simulink model "OVF2D"  (R2022b)
settings: Solver=FixedStepAuto  StartTime=0.0  StopTime=15  FixedStep=ts  MaxStep=0.6  RelTol=1e-3
values from neighbouring files (symbols this model uses):
  N = 4    [OVFMain.m]
  p_obstacle = [2,3;3,7;7.5,5.5]    [OVFMain.m]
  p_target = [9,10;3,10;6,10;0,10]    [OVFMain.m]
  ra = 0.6    [OVFMain.m]
  ro = [1.3;1.4;1.8]    [OVFMain.m]
  rs = 0.4    [OVFMain.m]
  v_max = 2    [OVFMain.m]
  v_max1 = 20    [OVFMain.m]
libraries: aerolibanimutils x1
settings Model: Creator=51078  LastModifiedBy=51078
settings SolverCC: AlgebraicLoopSolver=TrustRegion
settings DataIOCC: ReturnWorkspaceOutputs=off
settings DebuggingCC: UnconnectedInputMsg=warning  UnconnectedOutputMsg=warning  UnconnectedLineMsg=warning  SFMachineParentedDataDiag=warning  ArithmeticOperatorsInVariantConditions=warning
settings ModelReferenceCC: EnableRefExpFcnMdlSchedulingChecks=on
settings SFSimCC: SimUseLocalCustomCode=off  CustomCodeUndefinedFunction=UseInterfaceOnly
settings RTWCC: RTWUseLocalCustomCode=off  DLArmComputeVersion=19.05
settings CodeAppCC: StateflowObjectComments=on

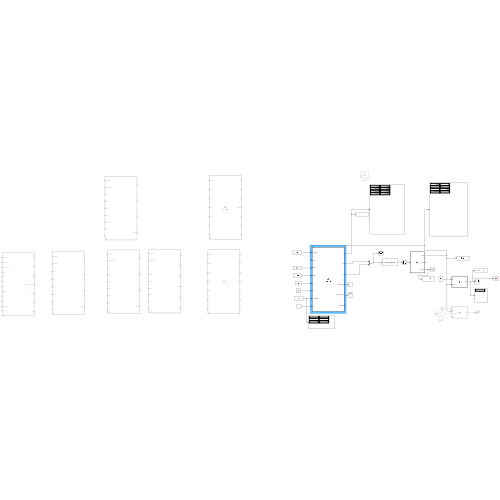
[thumbnail: Simulink's stored preview of the top-level diagram]
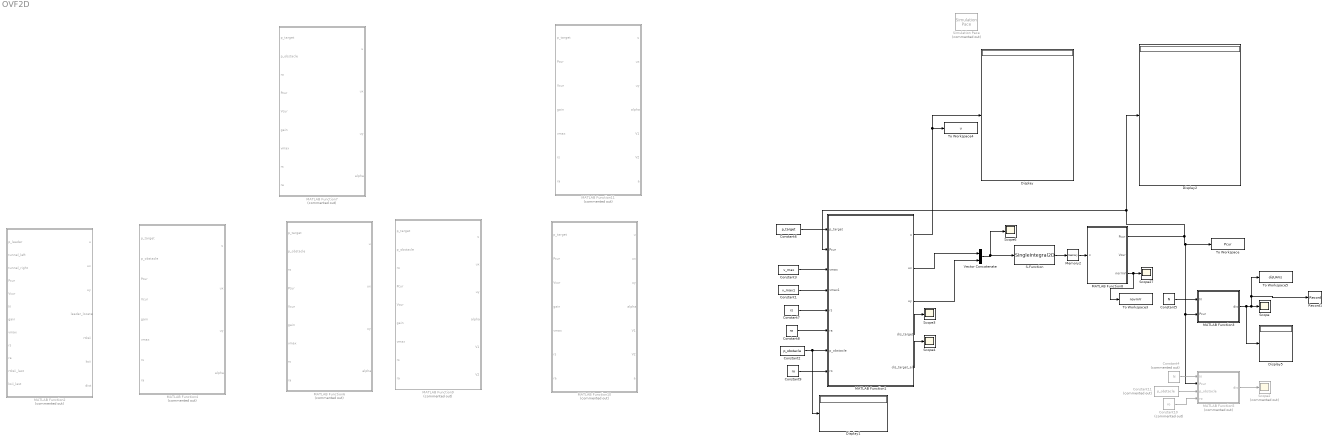
== system OVF2D ==
  Constant1 : Constant  Value=v_max1
  Constant10 : Constant  Commented=on  Value=ro
  Constant11 : Constant  Commented=on  Value=p_obstacle
  Constant2 : Constant  Value=p_obstacle
  Constant3 : Constant  Value=v_max
  Constant4 : Constant  Commented=on  Value=N
  Constant5 : Constant  Value=N
  Constant6 : Constant  Value=p_target
  Constant7 : Constant  Value=rs
  Constant8 : Constant  Value=ra
  Constant9 : Constant  Value=ro
  Display{,1..2,5} (4 alike) : Display
  MATLAB Function1 : MATLAB Function  TreatAsAtomicUnit=on
  MATLAB Function10 : MATLAB Function  Commented=on  TreatAsAtomicUnit=on
  MATLAB Function11 : MATLAB Function  Commented=on  TreatAsAtomicUnit=on
  MATLAB Function2 : MATLAB Function  Commented=on  TreatAsAtomicUnit=on
  MATLAB Function3 : MATLAB Function  TreatAsAtomicUnit=on
  MATLAB Function4 : MATLAB Function  Commented=on  TreatAsAtomicUnit=on
  MATLAB Function5 : MATLAB Function  Commented=on  TreatAsAtomicUnit=on
  MATLAB Function6 : MATLAB Function  Commented=on  TreatAsAtomicUnit=on
  MATLAB Function7 : MATLAB Function  Commented=on  TreatAsAtomicUnit=on
  MATLAB Function8 : MATLAB Function  TreatAsAtomicUnit=on
  MATLAB Function9 : MATLAB Function  Commented=on  TreatAsAtomicUnit=on
  Memory2 : Memory
  Record1 : Record  FileSettingsInternal="{\"entries\":[{\"content\":{\"excelSettings\":{\"content\":{},\"type\":\"Streamout.ExcelSettings\"}},\"type\":\"Streamout.FileSettingStorage\",\"uuid\":\"113e7f0b-c50f-4f8c-84db-ec7da5fa2ec4\"}],\"packageUris\":[\"http://schema.mathworks.com/mf0/streamout_blocks/R2020a\"],\"version\":\"1.0\"}"  Layout=[1 1]  SignalsInternal="{\"entries\":[{\"content\":{\"signals\":[{\"content\":{\"blockPath\":[\"OVF2D/Record1\"],\"channel\":[],\"dimensions\":[1],\"domain\":\"OVF2D/Record1\",\"lineColor\":\"#d95319\",\"plots\":[],\"port\":1,\"sid\":[\"\"],\"signalID\":16,\"signalName\":\"MATLAB Function3\"},\"type\":\"RecordBlkView.Signal\",\"uuid\":\"cb360406-dc3a-4a23-b0a4-c1b09b6a15ae\"}]},\"type\":\"RecordBlkView.InputSignals\",\"uuid\":\"8c052846-9eb7-4e55-9645-09fc1fafe585\"}],\"packageUris\":[\"http://schema.mathworks.com/mf0/streamout_blocks/R2020a\"],\"version\":\"1.0\"}"  VisualizationBindings="{\"sparklinesplugin\":{\"info\":[{\"bindingParametersList\":[],\"subplotID\":1}]}}"
  S-Function : S-Function  FunctionName=SingleIntegral2D  SFunctionDeploymentMode=off  EnableBusSupport=off
  Scope{,3..4,6,27} (5 alike) : Scope
  Scope2 : Scope  Commented=on
  Simulation Pace : aerolibanimutils/Simulation Pace  Commented=on  SimulationPace=1  SleepMode=MATLAB Thread  OutputPaceError=off  SampleTime=0.01
  To Workspace : ToWorkspace  VariableName=Pcur  SaveFormat=Timeseries  SampleTime=-1
  To Workspace3 : ToWorkspace  VariableName=novmV  SaveFormat=Timeseries  SampleTime=-1
  To Workspace4 : ToWorkspace  VariableName=u  SaveFormat=Timeseries  SampleTime=-1
  To Workspace5 : ToWorkspace  VariableName=disUAVs  SaveFormat=Timeseries  SampleTime=-1
  Vector Concatenate : Concatenate
  wires:
  Constant3/1 -> MATLAB Function1/3(vmax)
  Constant7/1 -> MATLAB Function1/5(rs)
  Constant8/1 -> MATLAB Function1/6(ra)
  MATLAB Function1/1(u) -> Display/1, To Workspace4/1
  Constant5/1 -> MATLAB Function3/1(N)
  MATLAB Function3/1(dis) -> Display5/1, Scope/1, Record1/1, To Workspace5/1
  Constant6/1 -> MATLAB Function1/1(p_target)
  MATLAB Function1/2(ux) -> Vector Concatenate/1
  MATLAB Function1/3(uy) -> Vector Concatenate/2
  MATLAB Function8/3(normV) -> To Workspace3/1, Scope27/1
  MATLAB Function8/1(Pcur) -> MATLAB Function5/2(Pcur), MATLAB Function3/2(Pcur), To Workspace/1, Display2/1, MATLAB Function1/2(Pcur)
  S-Function/1 -> Memory2/1
  Constant4/1 -> MATLAB Function5/1(N)
  MATLAB Function5/1(dis) -> Scope2/1
  Constant10/1 -> MATLAB Function5/4(ro)
  Constant11/1 -> MATLAB Function5/3(p_obstacle)
  MATLAB Function1/4(dis_target) -> Scope3/1
  Vector Concatenate/1 -> Scope6/1, S-Function/1
  Memory2/1 -> MATLAB Function8/1(x)
  Constant1/1 -> MATLAB Function1/4(vmax1)
  Constant2/1 -> Display1/1, MATLAB Function1/7(p_obstacle)
  Constant9/1 -> MATLAB Function1/8(ro)
  MATLAB Function1/5(dis_target_all) -> Scope4/1

== matlab function OVF2D/MATLAB Function6 ==
  data: p_target input; p_obstacle input; ro input; u output size=[N,2]; ux output size=[N,1]; uy output size=[N,1]; Pcur input; Vcur input; gain input; vmax input; rs input; ra input; alpha output
function [u,ux,uy,alpha]  = mytunnel(p_target,p_obstacle,ro,Pcur,Vcur,gain,vmax,rs,ra)
N=1;

e1=zeros(N,2);
V1=zeros(N,2);
V2=zeros(N,2);
V3=zeros(N,2);
V=zeros(N,2);

u=zeros(N,2);
ux=zeros(N,1);
uy=zeros(N,1);
OVF=2*ones(N,1);
alpha=zeros(N,1);

k1=1;
k2=40;
v2=zeros(N,2);
for i=1:N
    v_line=vmax;
    e1(i,:) = (p_target(i,:)-(Pcur(i,:)+1/gain*Vcur(i,1:2)))/norm(p_target(i,:)-(Pcur(i,:)+1/gain*Vcur(i,1:2)))*(v_line);
    V1(i,:) = mysat(k1*e1(i,:),vmax);
    
    for j=1:N
        if i~=j
            em = 0;
            ksimil = (Pcur(i,1:2) - Pcur(j,1:2)) + 1/gain*(Vcur(i,1:2) - Vcur(j,1:2));
            bil = k2*dmysigma2(norm(ksimil),2*rs,rs+ra,em);
            v2(i,:) = v2(i,:) + bil*(ksimil/norm(ksimil));
        end
    end
    
    for k=1:length(ro)
        em = 0;
        ksimik = (Pcur(i,1:2) - p_obstacle(k,1:2)) + 1/gain*(Vcur(i,1:2));
        bil = k2*dmysigma2(norm(ksimik),rs+ro(i),ro(i)+ra,em);
        v2(i,:) = v2(i,:) + bil*(ksimik/norm(ksimik));       
    end
    if isnan(v2(i,1)) || isnan(v2(i,2))
        v2(i,:)=[0,0];
    end
    
    
    
    ksiwp=(p_target(i,:)-(Pcur(i,:)+1/gain*Vcur(i,1:2)))/norm(p_target(i,:)-(Pcur(i,:)+1/gain*Vcur(i,1:2)));
    Ai = ksiwp'*ksiwp;    
    a=dot(v2(i,:),ksiwp)/(norm(v2(i,:))*norm(ksiwp));
    costheta1=-2/sqrt(5);
    costheta2=(norm(V1(i,:))-sqrt(5*norm(V1(i,:))^2+4*norm(v2(i,:))^2))/(2*norm(v2(i,:)));
    alpha(i)=mysigma3(a,costheta2,costheta1);
%     if a>0
%         alpha(i)=0;
%     end
     V2(i,:) = ((eye(2)-alpha(i)*Ai)*v2(i,:)')';

    % V2(i,:)=v2(i,:);
     
    if isnan(V2(i,1)) || isnan(V2(i,2))
        V2(i,:)=[0,0];
    end
    
    V(i,:)=mysat(V1(i,:)+V2(i,:),vmax);
end


u=V;
ux = u(:,1);
uy = u(:,2);

== matlab function OVF2D/MATLAB Function7 ==
  data: p_target input; p_obstacle input; ro input; u output size=[N,2]; ux output size=[N,1]; uy output size=[N,1]; Pcur input; Vcur input; gain input; vmax input; rs input; ra input; alpha output
function [u,ux,uy,alpha]  = mytunnel(p_target,p_obstacle,ro,Pcur,Vcur,gain,vmax,rs,ra)
N=1;

e1=zeros(N,2);
V1=zeros(N,2);
V2=zeros(N,2);
V3=zeros(N,2);
V=zeros(N,2);

u=zeros(N,2);
ux=zeros(N,1);
uy=zeros(N,1);
OVF=2*ones(N,1);
alpha=zeros(N,1);

k1=1;
k2=4;
v2=zeros(N,2);
for i=1:N
    v_line=vmax;
    e1(i,:) = (p_target(i,:)-(Pcur(i,:)+1/gain*Vcur(i,1:2)))/norm(p_target(i,:)-(Pcur(i,:)+1/gain*Vcur(i,1:2)))*(v_line);
    V1(i,:) = mysat(k1*e1(i,:),vmax);
    
    for j=1:N
        if i~=j
            em = 0;
            ksimil = (Pcur(i,1:2) - Pcur(j,1:2)) + 1/gain*(Vcur(i,1:2) - Vcur(j,1:2));
            bil = k2*dmysigma2(norm(ksimil),2*rs,rs+ra,em);
            v2(i,:) = v2(i,:) + bil*(ksimil/norm(ksimil));
        end
    end
    
    for k=1:length(ro)
        em = 0;
        ksimik = (Pcur(i,1:2) - p_obstacle(k,1:2)) + 1/gain*(Vcur(i,1:2));
        
%         bil = k2*dmysigma2(norm(ksimik),rs+ro(i),ro(i)+ra,em);
%         v2(i,:) = bil*(ksimik/norm(ksimik));     

        v2(i,:) = k2*norm((Pcur(i,:)+1/gain*Vcur(i,1:2))-p_target(i,:))^2*dmysigma2(norm(ksimik),rs+ro(i),ro(i)+ra,em)*(ksimik/norm(ksimik))...
            +mysigma2(norm(ksimik),rs+ro(i),ro(i)+ra,em)*2*(p_target(i,:)-(Pcur(i,:)+1/gain*Vcur(i,1:2)));     
        
        ksiwp=(p_target(i,:)-(Pcur(i,:)+1/gain*Vcur(i,1:2)))/norm(p_target(i,:)-(Pcur(i,:)+1/gain*Vcur(i,1:2)));
        Ai = ksiwp'*ksiwp;
        a=dot(v2(i,:),ksiwp)/(norm(v2(i,:))*norm(ksiwp));
        costheta1=-2/sqrt(5);
        costheta2=(norm(V1(i,:))-sqrt(5*norm(V1(i,:))^2+4*norm(v2(i,:))^2))/(2*norm(v2(i,:)));
        alpha(i)=mysigma3(a,costheta2,costheta1);
        %     if a>0
        %         alpha(i)=0;
        %     end
%         V2(i,:) = V2(i,:)+((eye(2)-alpha(i)*Ai)*v2(i,:)')';
         V2(i,:) = V2(i,:)+v2(i,:);

    end
    if isnan(V2(i,1)) || isnan(V2(i,2))
        V2(i,:)=[0,0];
    end
    
    V(i,:)=mysat(V1(i,:)+V2(i,:),vmax);
end


u=V;
ux = u(:,1);
uy = u(:,2);

== matlab function OVF2D/MATLAB Function2 ==
  data: p_leader input; tunnel_left input; u output size=[20,2]; ux output size=[20,1]; uy output size=[20,1]; tunnel_right input; Pcur input; Vcur input; N input; gain input; vmax input; leader_locate output; rs input; ra input; rtksii_last input; ksii_last input; rtksii output size=[20,1]; ksii output size=[20,2]; dist output
function [u,ux,uy,leader_locate,rtksii,ksii,dist]  = mytunnel(p_leader,tunnel_left,tunnel_right,Pcur,Vcur,N,gain,vmax,rs,ra,rtksii_last,ksii_last)

leader_locate=zeros(20,1);
for i=1:N
    dis_leader_min=10^8;
    for j=1:length(p_leader(:,1))
        dis_leader=norm(Pcur(i,:)-p_leader(j,:));
        if dis_leader < dis_leader_min
            leader_locate(i)=j;
            dis_leader_min=dis_leader;
        end
    end
end

nc=zeros(length(tunnel_left(:,1)),2);
for i=1:length(tunnel_left(:,1))
    rot=[0 -1;1 0]; %逆时针90度
    C=rot*(tunnel_right(i,:)-tunnel_left(i,:))';
    nc(i,:)=-(C/norm(C))';
end

e1=zeros(N,2);
V1=zeros(N,2);
V2=zeros(N,2);
V3=zeros(N,2);
V=zeros(N,2);

u=zeros(20,2);
ux=zeros(20,1);
uy=zeros(20,1);

rtksii=zeros(20,1);
ksiti=zeros(20,2);
ksii=zeros(20,2);
pti=zeros(20,2);

dis=10^5;
dist=10^5;


rs1=rs;
v_line=0;
for i=1:N
    if leader_locate(i)~=0
%         if i>=1 && i<=5
%             v_line=vmax;
%         elseif i>=6 && i<=10
%             v_line=vmax-0.7;
%         elseif i>=11 && i<=15
%             v_line=vmax-1.4;
%         elseif i>=16 && i<=20
%             v_line=vmax-2.1;
%         end
        v_line=vmax;
        
        %v_line=0.5*vmax;
        k1=1;
        e1(i,:) = nc(leader_locate(i),:)*(v_line);
        V1(i,:) = -mysat(k1*e1(i,:),vmax);
        
        et=10^(-1);e = 0.000001;
        k3=1;
        mksii=0.5*(tunnel_left(leader_locate(i),:)+tunnel_right(leader_locate(i),:));
        ksii(i,:) = Pcur(i,1:2) + 1/gain*Vcur(i,1:2);
        ksiti(i,:) = Pcur(i,1:2) + 1/gain*Vcur(i,1:2) - mksii;
        rtksii(i)=0.5*norm(tunnel_left(leader_locate(i),:)-tunnel_right(leader_locate(i),:));
        
        pti(i,:)= Pcur(i,1:2) - mksii;
        disti =  rtksii(i) - norm(pti(i,:));
        if disti<dist
            dist=disti;
        end
        
        temp_t=(rtksii(i)-rs1)-norm(ksiti(i,:))*mys((rtksii(i)-rs1)/(norm(ksiti(i,:))+et),e);
        dVtidksiti=(-k3*dmysigma(rtksii(i)-norm(ksiti(i,:)),rs1,ra)*temp_t+k3*mysigma(rtksii(i)-norm(ksiti(i,:)),rs1,ra)*(mys((rtksii(i)-rs1)/(norm(ksiti(i,:))+et),e)-norm(ksiti(i,:))*(rtksii(i)-rs1)/((norm(ksiti(i,:))+et)^2)*dmys((rtksii(i)-rs1)/(norm(ksiti(i,:))+et),e)))/(temp_t^2);
        dVtidrtksii=(k3*dmysigma(rtksii(i)-norm(ksiti(i,:)),rs1,ra)*temp_t-k3*mysigma(rtksii(i)-norm(ksiti(i,:)),rs1,ra)*(1-(norm(ksiti(i,:))/(norm(ksiti(i,:))+et))*dmys((rtksii(i)-rs1)/(norm(ksiti(i,:))+et),e)))/(temp_t^2);
        if ksii(i,1)-ksii_last(i,1)==0 || ksii(i,2)-ksii_last(i,2)==0
            drtpdksii=[0,0];
        else
            drtpdksii=[(rtksii(i)-rtksii_last(i))/(ksii(i,1)-ksii_last(i,1)),(rtksii(i)-rtksii_last(i))/(ksii(i,2)-ksii_last(i,2))];
        end
        ci=dVtidksiti*ksiti(i,:)/norm(ksiti(i,:))+dVtidrtksii*drtpdksii;
        
        un=ksiti(i,:)-(dot(ksiti(i,:),nc(leader_locate(i),:))*nc(leader_locate(i),:));
        V3(i,:)=-(un/norm(un))*dot(un/norm(un),ci);
        if isnan(V3(i,1)) || isnan(V3(i,2))
            V3(i,:)=[0,0];
        end
    end
    
    for j=1:N
        if i~=j
            k2 = 1; e = 0.000001;
            ksimil = (Pcur(i,1:2) - Pcur(j,1:2)) + 1/gain*(Vcur(i,1:2) - Vcur(j,1:2));
            temp = (1+e)*norm(ksimil) - (2*rs)*mys(norm(ksimil)/(2*rs),e);
            bil = k2*dmysigma(norm(ksimil),2*rs,rs+ra)/temp ...
                - k2*mysigma(norm(ksimil),2*rs,rs+ra)*((1+e)-dmys(norm(ksimil)/(2*rs),e))/(temp^2);
            V2(i,:) = V2(i,:)- bil*(ksimil/norm(ksimil));
            if isnan(V2(i,1)) || isnan(V2(i,2))
                V2(i,:)=[0,0];
            end
            disij=norm(Pcur(i,1:2) - Pcur(j,1:2));
            if disij<dis
                dis=disij;
            end
        end
    end
    V(i,:)=mysat(V1(i,:)+V2(i,:)+V3(i,:),vmax);
end
% V11=[V1(1,1:2);V1(2,1:2);V1(3,1:2);V1(4,1:2)];
% V21=[V2(1,1:2);V2(2,1:2);V2(3,1:2);V2(4,1:2)];
% V31=[V3(1,1:2);V3(2,1:2);V3(3,1:2);V3(4,1:2)];



u = [V(1,1:2);V(2,1:2);V(3,1:2);V(4,1:2);V(5,1:2);V(6,1:2);V(7,1:2);V(8,1:2);V(9,1:2);V(10,1:2);V(11,1:2);V(12,1:2);V(13,1:2);V(14,1:2);V(15,1:2);V(16,1:2);V(17,1:2);V(18,1:2);V(19,1:2);V(20,1:2)];
ux = u(:,1);
uy = u(:,2);

== matlab function OVF2D/MATLAB Function9 ==
  data: p_target input; p_obstacle input; ro input; u output size=[N,2]; ux output size=[N,1]; uy output size=[N,1]; Pcur input; Vcur input; gain input; vmax input; rs input; ra input; alpha output; V1 output; V2 output
function [u,ux,uy,alpha,V1,V2]  = mytunnel(p_target,p_obstacle,ro,Pcur,Vcur,gain,vmax,rs,ra)
tic
N=1;

e1=zeros(N,2);
V1=zeros(N,2);
V2=zeros(N,2);
V3=zeros(N,2);
V=zeros(N,2);

u=zeros(N,2);
ux=zeros(N,1);
uy=zeros(N,1);
OVF=2*ones(N,1);
alpha=zeros(N,1);

k1=1;
k2=4;
v2=zeros(N,2);
for i=1:N
    v_line=vmax;
    e1(i,:) = (p_target(i,:)-(Pcur(i,:)+1/gain*Vcur(i,1:2)))/norm(p_target(i,:)-(Pcur(i,:)+1/gain*Vcur(i,1:2)))*(v_line);
    V1(i,:) = mysat(k1*e1(i,:),vmax);
    
    for j=1:N
        if i~=j
            em = 0;
            ksimil = (Pcur(i,1:2) - Pcur(j,1:2)) + 1/gain*(Vcur(i,1:2) - Vcur(j,1:2));
            bil = k2*dmysigma2(norm(ksimil),2*rs,rs+ra,em);
            v2(i,:) = v2(i,:) + bil*(ksimil/norm(ksimil));
        end
    end
    
    for k=1:length(ro)
        em = 0;
        ksimik = (Pcur(i,1:2) - p_obstacle(k,1:2)) + 1/gain*(Vcur(i,1:2));
        
        bil = k2*dmysigma2(norm(ksimik),rs+ro(i),ro(i)+ra,em);
        v2(i,:) = bil*(ksimik/norm(ksimik));     
       
        ksiwp=(p_target(i,:)-(Pcur(i,:)+1/gain*Vcur(i,1:2)))/norm(p_target(i,:)-(Pcur(i,:)+1/gain*Vcur(i,1:2)));
        Ai = ksiwp'*ksiwp;
        a=dot(v2(i,:),ksiwp)/(norm(v2(i,:))*norm(ksiwp));
        costheta1=-2/sqrt(5);
        costheta2=(norm(V1(i,:))-sqrt(5*norm(V1(i,:))^2+4*norm(v2(i,:))^2))/(2*norm(v2(i,:)));
        alpha(i)=mysigma3(a,costheta2,costheta1);
        %     if a>0
        %         alpha(i)=0;
        %     end
        
        V2(i,:) = V2(i,:)+((eye(2)-alpha(i)*Ai)*v2(i,:)')';
         %V2(i,:) = V2(i,:)+((eye(2)-Ai)*v2(i,:)')';

        %V2(i,:) = V2(i,:)+v2(i,:);

    end
    if isnan(V2(i,1)) || isnan(V2(i,2))
        V2(i,:)=[0,0];
    end
    
    V(i,:)=mysat(V1(i,:)+V2(i,:),vmax);
end


u=V;
ux = u(:,1);
uy = u(:,2);
toc

== matlab function OVF2D/MATLAB Function10 ==
  data: p_target input; u output size=[N,2]; ux output size=[N,1]; uy output size=[N,1]; Pcur input; Vcur input; gain input; vmax input; rs input; ra input; alpha output; V1 output; V2 output; a output
function [u,ux,uy,alpha,V1,V2,a]  = mytunnel(p_target,Pcur,Vcur,gain,vmax,rs,ra)
% p_obstacle=p_obstacle';
% p_target=p_target';

N=4;
a=zeros(N,1);

e1=zeros(N,2);
V1=zeros(N,2);
V2=zeros(N,2);
V3=zeros(N,2);
V=zeros(N,2);

u=zeros(N,2);
ux=zeros(N,1);
uy=zeros(N,1);
OVF=2*ones(N,1);
alpha=zeros(N,1);

k1=1;
k2=100;
k3=3;
v2=zeros(N,2);
Ai=zeros(2,2);

for i=1:N
    v_line=vmax;
    e1(i,:) = (p_target(i,:)-Pcur(i,:))/norm(p_target(i,:)-Pcur(i,:))*(v_line);
%     e1(i,:) = (p_target(i,:)-Pcur(i,:));
    V1(i,:) = mysat(k1*e1(i,:),vmax);
    
    for j=1:N
        if i~=j
%             em = 0;
%             ksimil = (Pcur(i,1:2) - Pcur(j,1:2));
%             bil = k2*dmysigma2(norm(ksimil),2*rs,rs+ra,em);
%             v2(i,:) = v2(i,:) + bil*(ksimil/norm(ksimil));
            e = 0.000001;
            ksimil =  Pcur(i,1:2) - Pcur(j,1:2);
            temp = (1+e)*norm(ksimil) - (2*rs)*mys(norm(ksimil)/(2*rs),e);
            bil = k2*dmysigma(norm(ksimil),2*rs,rs+ra)/temp ...
                - k2*mysigma(norm(ksimil),2*rs,rs+ra)*((1+e)-dmys(norm(ksimil)/(2*rs),e))/(temp^2);
            v2(i,:)  = v2(i,:)  -  bil*(ksimil/norm(ksimil));
        end
    end
    
    
%     ksiwp=(p_target(i,:)-(Pcur(i,:)+1/gain*Vcur(i,1:2)))/norm(p_target(i,:)-(Pcur(i,:)+1/gain*Vcur(i,1:2)));
%     Ai = ksiwp'*ksiwp;
%     a=dot(v2(i,:),ksiwp)/(norm(v2(i,:))*norm(ksiwp));
%     costheta1=-2/sqrt(5);
%     costheta2=(norm(V1(i,:))-sqrt(5*norm(V1(i,:))^2+4*norm(v2(i,:))^2))/(2*norm(v2(i,:)));
%     alpha(i)=mysigma3(a,costheta2,costheta1);
%     if a>0
%         alpha(i)=0;
%     end
%     V2(i,:) = V2(i,:)+((eye(2)-alpha(i)*Ai)*v2(i,:)')';

    
     costheta=dot(V1(i,:) ,v2(i,:) )/(norm(V1(i,:) )*norm(v2(i,:) ));     
    if V1(i,1)*v2(i,2)-V1(i,2)*v2(i,1)>0 && costheta<0
        V2(i,:)= v2(i,:) + (norm(v2(i,:))/(sqrt(1-costheta^2)/-costheta))*(Rotation(-pi/2)*v2(i,:)'/norm(v2(i,:)))';
    elseif V1(i,1)*v2(i,2)-V1(i,2)*v2(i,1)<0 && costheta<0
        V2(i,:)= v2(i,:) + (norm(v2(i,:))/(sqrt(1-costheta^2)/-costheta))*(Rotation(pi/2)*v2(i,:)'/norm(v2(i,:)))';
    elseif costheta>=0
        V2(i,:)= v2(i,:) ;
    elseif V1(i,1)*v2(i,2)-V1(i,2)*v2(i,1)==0 && costheta<0
        V2(i,:)= v2(i,:)+ (Rotation(pi/2)*v2(i,:)')';
    else
        V2(i,:)=zeros(1,2);
    end
    


    Ai = V1(i,:)'*V1(i,:)/(norm(V1(i,:))^2);
    costheta1=cos(deg2rad(125));
    costheta2=-sqrt(2)/2;
    alpha(i)=mysigma3(costheta,costheta2,costheta1);
    if costheta>0
        alpha(i)=0;
    end

    a(i)=V1(i,1)*v2(i,2)-V1(i,2)*v2(i,1);
    if V1(i,1)*v2(i,2)-V1(i,2)*v2(i,1)>0
        V3(i,:)= ((eye(2)-alpha(i)*Ai)*v2(i,:)')' + dmysigma2(costheta,-1,costheta2,0)*(Rotation(-pi/2)*v2(i,:)')';
    elseif V1(i,1)*v2(i,2)-V1(i,2)*v2(i,1)<0
        V3(i,:)= ((eye(2)-alpha(i)*Ai)*v2(i,:)')' + dmysigma2(costheta,-1,costheta2,0)*(Rotation(pi/2)*v2(i,:)')';
    elseif V1(i,1)*v2(i,2)-V1(i,2)*v2(i,1)==0 && costheta>0
        V3(i,:)= ((eye(2)-alpha(i)*Ai)*v2(i,:)')';
    elseif V1(i,1)*v2(i,2)-V1(i,2)*v2(i,1)==0 && costheta<0
        V3(i,:)= ((eye(2)-alpha(i)*Ai)*v2(i,:)')'+ dmysigma2(costheta,-1,costheta2,0)*(Rotation(pi/2)*v2(i,:)')';
    else
        V3(i,:)=zeros(1,2);
    end

%     V(i,:)=mysat(V1(i,:)+V3(i,:),vmax);
    V(i,:)=vmax*(V1(i,:)+V3(i,:))/norm(V1(i,:)+V3(i,:));

    if isnan(V(i,1)) || isnan(V(i,2))
        V(i,:)=[0,0];
    end
end


u=V;
ux = u(:,1);
uy = u(:,2);

== matlab function OVF2D/MATLAB Function11 ==
  data: p_target input; u output size=[N,2]; ux output size=[N,1]; uy output size=[N,1]; Pcur input; Vcur input; gain input; vmax input; rs input; ra input; alpha output; V1 output; V2 output; a output
function [u,ux,uy,alpha,V1,V2,a]  = mytunnel(p_target,Pcur,Vcur,gain,vmax,rs,ra)
% p_obstacle=p_obstacle';
% p_target=p_target';

N=4;
a=zeros(N,1);

e1=zeros(N,2);
V1=zeros(N,2);
V2=zeros(N,2);
V3=zeros(N,2);
V=zeros(N,2);

u=zeros(N,2);
ux=zeros(N,1);
uy=zeros(N,1);
OVF=2*ones(N,1);
alpha=zeros(N,1);

k1=1;
k2=100;
k3=3;
v2=zeros(N,2);
Ai=zeros(2,2);

for i=1:N
    v_line=vmax;
    e1(i,:) = (p_target(i,:)-Pcur(i,:))/norm(p_target(i,:)-Pcur(i,:))*(v_line);
%     e1(i,:) = log(p_target(i,:)-Pcur(i,:));
    V1(i,:) = k1*e1(i,:);
    
    for j=1:N
        if i~=j
%             em = 0;
%             ksimil = (Pcur(i,1:2) - Pcur(j,1:2));
%             bil = k2*dmysigma2(norm(ksimil),2*rs,rs+ra,em);
%             v2(i,:) = v2(i,:) + bil*(ksimil/norm(ksimil));
%             e = 0.000001;
%             ksimil =  Pcur(i,1:2) - Pcur(j,1:2);
%             temp = (1+e)*norm(ksimil) - (2*rs)*mys(norm(ksimil)/(2*rs),e);
%             bil = k2*dmysigma(norm(ksimil),2*rs,rs+ra)/temp ...
%                 - k2*mysigma(norm(ksimil),2*rs,rs+ra)*((1+e)-dmys(norm(ksimil)/(2*rs),e))/(temp^2);
%             v2(i,:)  = v2(i,:)  -  bil*(ksimil/norm(ksimil));
                ksimil =  Pcur(i,1:2) - Pcur(j,1:2);
                bil=1/(norm(ksimil)-2*rs);
                v2(i,:)  = v2(i,:)  +  bil*(ksimil/norm(ksimil));
        end
    end
    V2(i,:)=v2(i,:);
    
%     ksiwp=(p_target(i,:)-(Pcur(i,:)+1/gain*Vcur(i,1:2)))/norm(p_target(i,:)-(Pcur(i,:)+1/gain*Vcur(i,1:2)));
%     Ai = ksiwp'*ksiwp;
%     a=dot(v2(i,:),ksiwp)/(norm(v2(i,:))*norm(ksiwp));
%     costheta1=-2/sqrt(5);
%     costheta2=(norm(V1(i,:))-sqrt(5*norm(V1(i,:))^2+4*norm(v2(i,:))^2))/(2*norm(v2(i,:)));
%     alpha(i)=mysigma3(a,costheta2,costheta1);
%     if a>0
%         alpha(i)=0;
%     end
%     V2(i,:) = V2(i,:)+((eye(2)-alpha(i)*Ai)*v2(i,:)')';

    
%      costheta=dot(V1(i,:) ,v2(i,:) )/(norm(V1(i,:) )*norm(v2(i,:) ));     
%     if V1(i,1)*v2(i,2)-V1(i,2)*v2(i,1)>0 && costheta<0
%         V2(i,:)= v2(i,:) + (norm(v2(i,:))/(sqrt(1-costheta^2)/-costheta))*(Rotation(-pi/2)*v2(i,:)'/norm(v2(i,:)))';
%     elseif V1(i,1)*v2(i,2)-V1(i,2)*v2(i,1)<0 && costheta<0
%         V2(i,:)= v2(i,:) + (norm(v2(i,:))/(sqrt(1-costheta^2)/-costheta))*(Rotation(pi/2)*v2(i,:)'/norm(v2(i,:)))';
%     elseif costheta>=0
%         V2(i,:)= v2(i,:) ;
%     elseif V1(i,1)*v2(i,2)-V1(i,2)*v2(i,1)==0 && costheta<0
%         V2(i,:)= v2(i,:)+ (Rotation(pi/2)*v2(i,:)')';
%     else
%         V2(i,:)=zeros(1,2);
%     end
%     
% 
% 
%     Ai = V1(i,:)'*V1(i,:)/(norm(V1(i,:))^2);
%     costheta1=cos(deg2rad(125));
%     costheta2=-sqrt(2)/2;
%     alpha(i)=mysigma3(costheta,costheta2,costheta1);
%     if costheta>0
%         alpha(i)=0;
%     end
% 
%     a(i)=V1(i,1)*v2(i,2)-V1(i,2)*v2(i,1);
%     if V1(i,1)*v2(i,2)-V1(i,2)*v2(i,1)>0
%         V3(i,:)= ((eye(2)-alpha(i)*Ai)*v2(i,:)')' + dmysigma2(costheta,-1,costheta2,0)*(Rotation(-pi/2)*v2(i,:)')';
%     elseif V1(i,1)*v2(i,2)-V1(i,2)*v2(i,1)<0
%         V3(i,:)= ((eye(2)-alpha(i)*Ai)*v2(i,:)')' + dmysigma2(costheta,-1,costheta2,0)*(Rotation(pi/2)*v2(i,:)')';
%     elseif V1(i,1)*v2(i,2)-V1(i,2)*v2(i,1)==0 && costheta>0
%         V3(i,:)= ((eye(2)-alpha(i)*Ai)*v2(i,:)')';
%     elseif V1(i,1)*v2(i,2)-V1(i,2)*v2(i,1)==0 && costheta<0
%         V3(i,:)= ((eye(2)-alpha(i)*Ai)*v2(i,:)')'+ dmysigma2(costheta,-1,costheta2,0)*(Rotation(pi/2)*v2(i,:)')';
%     else
%         V3(i,:)=zeros(1,2);
%     end

    V(i,:)=mysat(V1(i,:)+V2(i,:),vmax);
%     V(i,:)=vmax*(V1(i,:)+V2(i,:))/norm(V1(i,:)+V2(i,:));
%     V(i,:)=V1(i,:)+V2(i,:);

    if isnan(V(i,1)) || isnan(V(i,2))
        V(i,:)=[0,0];
    end
end


u=V;
ux = u(:,1);
uy = u(:,2);

== matlab function OVF2D/MATLAB Function3 ==
  data: dis output; N input; Pcur input
function dis = fcn(N, Pcur)
dis=10^5;
for i=1:N
    for j=1:N
        if i~=j
            disij=norm(Pcur(i,1:2) - Pcur(j,1:2));
            if disij<dis
                dis=disij;
            end
        end
    end
end

== matlab function OVF2D/MATLAB Function8 ==
  data: x input; Pcur output size=[N,2]; Vcur output size=[N,2]; normV output
function [Pcur,Vcur,normV] = fcn(x)
N=4;
Pcur=zeros(N,2);
Vcur=zeros(N,2);
normV=zeros(N,1);
for i=1:N
    Pcur(i,1)=x(i);
    Pcur(i,2)=x(i+N);
    Vcur(i,1)=x(i+2*N);
    Vcur(i,2)=x(i+3*N);
    normV(i)=norm(Vcur(i,:));
end
end

== matlab function OVF2D/MATLAB Function1 ==
  data: p_target input; u output size=[N,2]; ux output size=[N,1]; uy output size=[N,1]; Pcur input; vmax input; vmax1 input; rs input; ra input; dis_target output; dis_target_all output; p_obstacle input; ro input
function [u,ux,uy,dis_target,dis_target_all]  = OVF(p_target,Pcur,vmax,vmax1,rs,ra,p_obstacle,ro)
% p_obstacle=p_obstacle';
% p_target=p_target';

N=4;
item=3;

e1=zeros(N,2);
V1=zeros(N,2);
V2=zeros(N,2);
V=zeros(N,2);

u=zeros(N,2);
ux=zeros(N,1);
uy=zeros(N,1);
gamma=zeros(N,1);

k1=1;
k2=10;
v2=zeros(N,2);
v3=zeros(N,2);
v4=zeros(N,2);

Ai=zeros(2,2);

dis_target_all=zeros(N,1);
dis_target=10^5;

for i=1:N
    dis_target_all(i)=norm(Pcur(i,1:2)-p_target(i,:));
end
dis_target=max(dis_target_all);

for i=1:N
    v_line=vmax;
    e1(i,:) = (p_target(i,:)-Pcur(i,:))/norm(p_target(i,:)-Pcur(i,:))*(v_line);
    V1(i,:) = mysat(k1*e1(i,:),vmax);
    
    for j=1:N
        if i~=j
            e = 0.000001;
            ksimil =  Pcur(i,1:2) - Pcur(j,1:2);
            temp = (1+e)*norm(ksimil) - (2*rs)*mys(norm(ksimil)/(2*rs),e);
            bil = k2*dmysigma(norm(ksimil),2*rs,rs+ra)/temp ...
                - k2*mysigma(norm(ksimil),2*rs,rs+ra)*((1+e)-dmys(norm(ksimil)/(2*rs),e))/(temp^2);
            v3(i,:)  = v3(i,:)  -  bil*(ksimil/norm(ksimil));
        end
    end
    
    for j=1:length(p_obstacle(:,1))
        e = 0.000001;
        ksimil =  Pcur(i,1:2) - p_obstacle(j,1:2);
        temp = (1+e)*norm(ksimil) - (rs+ro(j))*mys(norm(ksimil)/(rs+ro(j)),e);
        bil = k2*dmysigma(norm(ksimil),rs+ro(j),ra+ro(j))/temp ...
            - k2*mysigma(norm(ksimil),rs+ro(j),ra+ro(j))*((1+e)-dmys(norm(ksimil)/(rs+ro(j)),e))/(temp^2);
        v4(i,:)  = v4(i,:)  -  bil*(ksimil/norm(ksimil));
    end
    
    v2(i,:)=v3(i,:)+ v4(i,:);
    alpha=(norm(V1(i,:))-sqrt(5*norm(V1(i,:))^2+4*norm(v2(i,:))^2))/(2*norm(v2(i,:)));
    beta=norm(V1(i,:))/vmax1-sqrt(norm(V1(i,:))^2*norm(v2(i,:))^2+4*vmax1*norm(V1(i,:))^2*norm(v2(i,:))+4*vmax1^2*norm(v2(i,:))^2)/(2*vmax1*norm(v2(i,:)));
    mu=0;
    if norm(v2(i,:))<vmax1
        mu=alpha;
    elseif norm(v2(i,:))>=vmax1
        mu=beta;
    end
    
    Ai = (V1(i,:)/norm(V1(i,:)))'*(V1(i,:)/norm(V1(i,:)));
    chi=dot(v2(i,:),V1(i,:))/(norm(v2(i,:))*norm(V1(i,:)));
    gamma(i)=mysigma3(chi,mu,-2/sqrt(5)*mu/alpha);
    
    if item==1
        V2(i,:)=v2(i,:);
    elseif item==2
        V2(i,:)=mysat(v2(i,:),vmax1);
    elseif item==3
        if chi>0
            gamma(i)=0;
        end
        V2(i,:)=((eye(2)-gamma(i)*Ai)*mysat(v2(i,:),vmax1)')';
    end
    
    if isnan(V1(i,1))
        V1(i,:)=[0,0];
    end
    if isnan(V2(i,2))
        V2(i,:)=[0,0];
    end
    V(i,:)=mysat(V1(i,:)+V2(i,:),vmax);
end


u=V;
ux = u(:,1);
uy = u(:,2);

== matlab function OVF2D/MATLAB Function4 ==
  data: p_target input; p_obstacle input; u output size=[N,2]; ux output size=[N,1]; uy output size=[N,1]; Pcur input; Vcur input; gain input; vmax input; rs input; ra input; alpha output
function [u,ux,uy,alpha]  = mytunnel(p_target,p_obstacle,Pcur,Vcur,gain,vmax,rs,ra)
N=5;

e1=zeros(N,2);
V1=zeros(N,2);
V2=zeros(N,2);
V3=zeros(N,2);
V=zeros(N,2);

u=zeros(N,2);
ux=zeros(N,1);
uy=zeros(N,1);
OVF=2*ones(N,1);
alpha=zeros(N,1);

k1=1;
k2=4;
% ksimil=zeros(N,2);
v2=zeros(N,2);
for i=1:N
    v_line=vmax;
    e1(i,:) = (p_target(i,:)-(Pcur(i,:)+1/gain*Vcur(i,1:2)))/norm(p_target(i,:)-(Pcur(i,:)+1/gain*Vcur(i,1:2)))*(v_line);
    V1(i,:) = mysat(k1*e1(i,:),vmax);
    
    for j=1:N
        if i~=j
            em = 0;
            ksimil = (Pcur(i,1:2) - Pcur(j,1:2)) + 1/gain*(Vcur(i,1:2) - Vcur(j,1:2));
            bil = k2*dmysigma2(norm(ksimil),2*rs,rs+ra,em);
            v2(i,:) = v2(i,:) + bil*(ksimil/norm(ksimil));
            if isnan(v2(i,1)) || isnan(v2(i,2))
                v2(i,:)=[0,0];
            end
        end
    end
    ksiwp=(p_target(i,:)-(Pcur(i,:)+1/gain*Vcur(i,1:2)))/norm(p_target(i,:)-(Pcur(i,:)+1/gain*Vcur(i,1:2)));
    
    Ai = ksiwp'*ksiwp;    
    a=dot(v2(i,:),ksiwp)/(norm(v2(i,:))*norm(ksiwp));
    costheta1=-2/sqrt(5);
    costheta2=(norm(V1(i,:))-sqrt(5*norm(V1(i,:))^2+4*norm(v2(i,:))^2))/(2*norm(v2(i,:)));
    alpha(i)=mysigma3(a,costheta2,costheta1);

%     a=acos(dot(v2(i,:),ksiwp)/(norm(v2(i,:))*norm(ksiwp)));
%     theta1=acos(-2/sqrt(5));
%     theta2=acos(mysat((norm(V1(i,:))-sqrt(5*norm(V1(i,:))^2+4*norm(v2(i,:))^2))/(2*norm(v2(i,:))),1));
%     alpha(i)=mysigma(a,theta1,theta2);

     V2(i,:) = ((eye(2)-alpha(i)*Ai)*v2(i,:)')';
%     V2(i,:) = ((eye(2)-Ai)*v2(i,:)')';
%    V2(i,:) = v2(i,:);  

%     if a>-2/sqrt(5)
%         V2(i,:) = ((eye(2)-Ai)*v2(i,:)')';
%         OVF(i)=1;
%     else
%         V2(i,:) = v2(i,:);
%         OVF(i)=0;
%     end

    if isnan(V2(i,1)) || isnan(V2(i,2))
        V2(i,:)=[0,0];
    end
    
    V(i,:)=mysat(V1(i,:)+V2(i,:),vmax);
end


u=V;
ux = u(:,1);
uy = u(:,2);

== matlab function OVF2D/MATLAB Function5 ==
  data: dis output; N input; Pcur input; p_obstacle input; ro input
function dis = fcn(N, Pcur,p_obstacle,ro)
dis=10^5;
for i=1:N
    for j=1:length(ro)
        disij=norm(Pcur(i,:) - p_obstacle(j,:));
        if disij<dis
            dis=disij;
        end
    end
end
